simulink model "controllo_disco_rigido"  (R2019b)
settings: Solver=VariableStepAuto  StartTime=0.0  StopTime=10.0  RelTol=1e-3
values from neighbouring files (symbols this model uses):
  b = 0.002    [controllo_disco_rigido.m]    (also in controllo_disco_rigido_baseWS.mat; controllo_disco_rigido_script.m; init_controllo_disco_rigido.m)
  delay = 0.3    [controllo_disco_rigido.m]    (also in controllo_disco_rigido_script.m)
  J = 0.001    [controllo_disco_rigido.m]    (also in controllo_disco_rigido_baseWS.mat; controllo_disco_rigido_script.m; init_controllo_disco_rigido.m)
  R1 = 100    [controllo_disco_rigido.m]    (also in controllo_disco_rigido_script.m = 10^(round((((Ed)+20*wd(end))/20)-1))/gsys(3))
  R1_n = 10000    [controllo_disco_rigido.m]    (also in controllo_disco_rigido_script.m = 35000)
  R2_den = [1 1400]    [controllo_disco_rigido.m]    (also in controllo_disco_rigido_script.m = s-R2_pole)
  R2_n_den = [1 1540 196000]    [controllo_disco_rigido.m]
  R2_n_num = [1 2]    [controllo_disco_rigido.m]
  R2_num = [1 2]    [controllo_disco_rigido.m]    (also in controllo_disco_rigido_script.m = s-R2_zero)
  ritardo = exp(-delay*s)    [controllo_disco_rigido.m]    (also in controllo_disco_rigido_script.m)
  y0 = 300    [controllo_disco_rigido.m]    (also in controllo_disco_rigido_script.m)
libraries: cstblocks x2
settings Model: Creator=Utente  LastModifiedBy=Utente

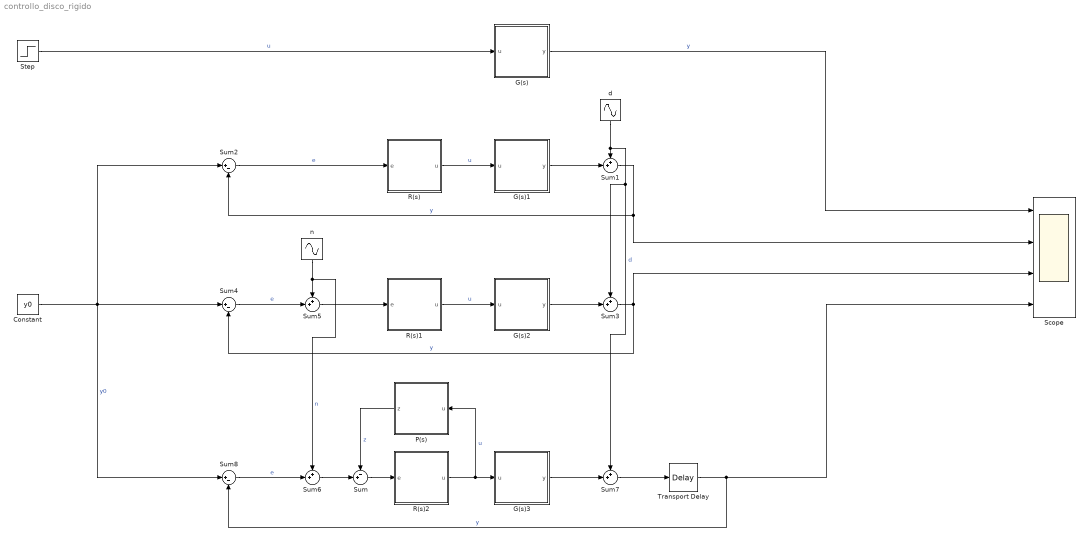
== system controllo_disco_rigido ==
  Constant : Constant  Value=y0
  G(s) : Subsystem
  G(s)1 : Subsystem
  G(s)2 : Subsystem
  G(s)3 : Subsystem
  P(s) : Subsystem
  R(s) : Subsystem
  R(s)1 : Subsystem
  R(s)2 : Subsystem
  Scope : Scope  NumInputPorts=4
  Step : Step  Time=0  SampleTime=0
  Sum : Sum  Inputs=-+|
  Sum{1,3,5..7} (5 alike) : Sum  Inputs=++|
  Sum2 : Sum  Inputs=|+-
  Sum4 : Sum  Inputs=|+-
  Sum8 : Sum  Inputs=|+-
  Transport Delay : TransportDelay  DelayTime=delay
  d : Sin  Frequency=[5]  SampleTime=0
  n : Sin  Frequency=[50]  SampleTime=0
  wires:
  G(s)/1(y) -> Scope/1  "y"
  Step/1 -> G(s)/1(u)  "u"
  Sum2/1 -> R(s)/1(e)  "e"
  R(s)/1(u) -> G(s)1/1(u)  "u"
  Sum1/1 -> Scope/2, Sum2/2  "y"
  G(s)1/1(y) -> Sum1/2
  Sum3/1 -> Scope/3, Sum4/2  "y"
  Sum4/1 -> Sum5/2  "e"
  Sum5/1 -> R(s)1/1(e)
  R(s)1/1(u) -> G(s)2/1(u)  "u"
  G(s)2/1(y) -> Sum3/2
  Sum/1 -> R(s)2/1(e)
  P(s)/1(z) -> Sum/1  "z"
  Sum7/1 -> Transport Delay/1
  Sum6/1 -> Sum/2
  G(s)3/1(y) -> Sum7/2
  Constant/1 -> Sum2/1, Sum8/1, Sum4/1  "y0"
  Transport Delay/1 -> Scope/4, Sum8/2  "y"
  Sum8/1 -> Sum6/2  "e"
  R(s)2/1(u) -> P(s)/1(u), G(s)3/1(u)  "u"
  n/1 -> Sum6/1, Sum5/1  "n"
  d/1 -> Sum7/1, Sum3/1, Sum1/1  "d"

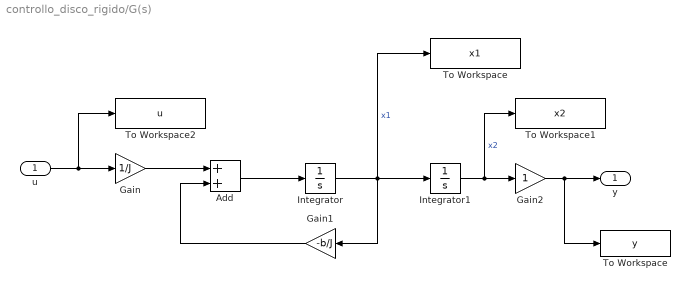
== system controllo_disco_rigido/G(s) ==
  u : Inport
  " To Workspace" : ToWorkspace  VariableName=y  SampleTime=-1
  Add : Sum
  Gain : Gain  Gain=1/J
  Gain1 : Gain  Gain=-b/J
  Gain2 : Gain
  Integrator : Integrator
  Integrator1 : Integrator
  To Workspace : ToWorkspace  VariableName=x1  SampleTime=-1
  To Workspace1 : ToWorkspace  VariableName=x2  SampleTime=-1
  To Workspace2 : ToWorkspace  VariableName=u  SampleTime=-1
  y : Outport
  wires:
  Integrator/1 -> To Workspace/1, Gain1/1, Integrator1/1  "x1"
  u/1 -> Gain/1, To Workspace2/1
  Add/1 -> Integrator/1
  Gain/1 -> Add/1
  Gain1/1 -> Add/2
  Integrator1/1 -> Gain2/1, To Workspace1/1  "x2"
  Gain2/1 -> " To Workspace"/1, y/1

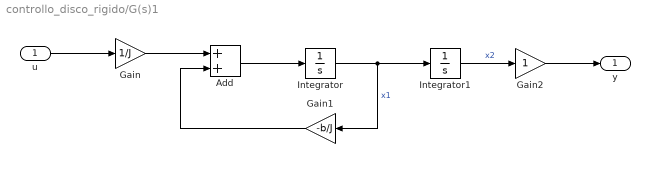
== system controllo_disco_rigido/G(s)1 ==
  u : Inport
  Add : Sum
  Gain : Gain  Gain=1/J
  Gain1 : Gain  Gain=-b/J
  Gain2 : Gain
  Integrator : Integrator
  Integrator1 : Integrator
  y : Outport
  wires:
  Integrator/1 -> Gain1/1, Integrator1/1  "x1"
  u/1 -> Gain/1
  Add/1 -> Integrator/1
  Gain/1 -> Add/1
  Gain1/1 -> Add/2
  Integrator1/1 -> Gain2/1  "x2"
  Gain2/1 -> y/1

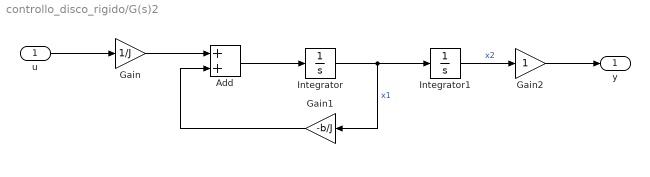
== system controllo_disco_rigido/G(s)2 ==
  u : Inport
  Add : Sum
  Gain : Gain  Gain=1/J
  Gain1 : Gain  Gain=-b/J
  Gain2 : Gain
  Integrator : Integrator
  Integrator1 : Integrator
  y : Outport
  wires:
  Integrator/1 -> Gain1/1, Integrator1/1  "x1"
  u/1 -> Gain/1
  Add/1 -> Integrator/1
  Gain/1 -> Add/1
  Gain1/1 -> Add/2
  Integrator1/1 -> Gain2/1  "x2"
  Gain2/1 -> y/1

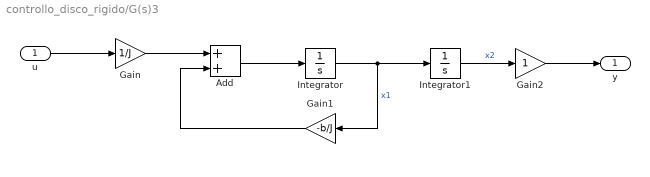
== system controllo_disco_rigido/G(s)3 ==
  u : Inport
  Add : Sum
  Gain : Gain  Gain=1/J
  Gain1 : Gain  Gain=-b/J
  Gain2 : Gain
  Integrator : Integrator
  Integrator1 : Integrator
  y : Outport
  wires:
  Integrator/1 -> Gain1/1, Integrator1/1  "x1"
  u/1 -> Gain/1
  Add/1 -> Integrator/1
  Gain/1 -> Add/1
  Gain1/1 -> Add/2
  Integrator1/1 -> Gain2/1  "x2"
  Gain2/1 -> y/1

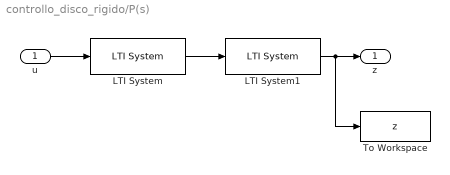
== system controllo_disco_rigido/P(s) ==
  u : Inport
  LTI System : cstblocks/LTI System  sys=sys_tf  IC=[]
  LTI System1 : cstblocks/LTI System  sys=1-ritardo  IC=[]
  To Workspace : ToWorkspace  VariableName=z  SampleTime=-1
  z : Outport
  wires:
  u/1 -> LTI System/1
  LTI System1/1 -> To Workspace/1, z/1
  LTI System/1 -> LTI System1/1

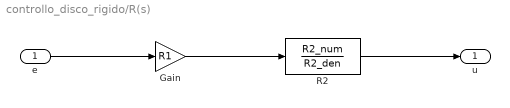
== system controllo_disco_rigido/R(s) ==
  e : Inport
  Gain : Gain  Gain=R1
  R2 : TransferFcn  Numerator=R2_num  Denominator=R2_den
  u : Outport
  wires:
  R2/1 -> u/1
  Gain/1 -> R2/1
  e/1 -> Gain/1

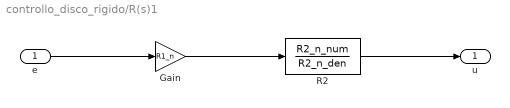
== system controllo_disco_rigido/R(s)1 ==
  e : Inport
  Gain : Gain  Gain=R1_n
  R2 : TransferFcn  Numerator=R2_n_num  Denominator=R2_n_den
  u : Outport
  wires:
  R2/1 -> u/1
  Gain/1 -> R2/1
  e/1 -> Gain/1

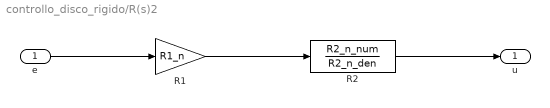
== system controllo_disco_rigido/R(s)2 ==
  e : Inport
  R1 : Gain  Gain=R1_n
  R2 : TransferFcn  Numerator=R2_n_num  Denominator=R2_n_den
  u : Outport
  wires:
  R1/1 -> R2/1
  e/1 -> R1/1
  R2/1 -> u/1
